simulink model "xPC_parker"  (Simulink 8.5)
settings: Solver=FixedStepDiscrete  StartTime=0.0  StopTime=inf  FixedStep=dts  RelTol=1e-3
InitFcn:
  | PARKER_DEPENDENCY
  | Parker_Multi_Axis_Init
  | Parker_ATI_Init
  | Parker_Home_Init
  | Parker_Davinci_Init
  | Parker_UDP_Init
  | Parker_LinIntPathPlan_Init
  | Parker_ScopeFormat_Init
  | Parker_magnetic_init
undefined symbols (not defined in the file): A, accel_filter_coeffs, ATI_torque_Nmm, B, counter_offset, DavinciFilterDen, DavinciFilterNum, DesiredPath, dt, dt_ENC, dt_trakstar, dts, dtudp, ENC_obs_filter_coeffs, encoder_counts, F, f_mag_desired_shape, filter_coeffs_bias, force_bias, forceDeadZone, FT_unbias_time, grav_vector, Home_in_TKbase, HOMING_dx, HOMING_num_joint, HOMING_tspan, HOMING_Vmov, inv_T, JOINT_Limits_Negative, JOINT_Limits_Postive, Kd, Ki_force, Kp, Kp_force, Kv_force, Low, N_acceleration, N_bias, N_ENC_obs_filter, N_obs_velocity, N_trakstar, N_velocity, Omega7IsLeftHanded, omni_scaling, PathPlanSpeed, pitch, quadrature_mode, R_FT2robot, R_omni, R_robot2TKbase, ResRateEpsilon, ResRateVelLimits, ResRateVelRatios, SafetyMargin, screw_pitch, torque_constant, trakstar_filter_coeffs, UDP_EN_Data2CMU, UDP_EN_DynAna, UDP_EN_VFRec ... (+6)
libraries: slrtlib x25, simulink x24, dspswit3 x15, xpcobsoletelib x15, xpcrtudplib x14, powerlib_meascontrol x3, xpcmeasurementcomputinglib x3, xpcconteclib x3
(part 2 of 3)

== system xPC_parker/Parker 404XR/Plant ==
  u : Inport
  "1STPORTB " : xpcmeasurementcomputinglib/Digital Input/PCI-DDA08 12   channel=[3 4 7]  port=C  chip=1  sampletime=dt  slot=-1
  CNT32-8M(PCI) Ch1 : xpcconteclib/Incremental Encoder/CNT32-8M(PCI)   Channel=1  OperationMode=2-phase Input Synchronous Clear Multiply by 4  DigitalFilter=No filtering  PulseInput=Differential line receiver input  Direction=Down in the clockwise direction/Up in the counterclockwise direction  InitialValue=counter_offset  LoadInitialValue=on  SampleTime=dt_ENC  PciSlot=-1  StartMethod=Model Start  StopMethod=Model Terminate  ZeroClearRising=off  ZeroClearFalling=off  ZeroClearMatch0=off  ZeroClearMatch1=off  PresetRising=off  PresetFalling=off  PresetMatch0=off  PresetMatch1=off  PresetValue=0  Match0Value=0  Match1Value=0  OutputSignalMatch0=off  OutputSignalMatch1=off  OutputSignalAbnormal=off  OutputSignalDigitalFilter=off  OutputSignalAlarm=off  OneShotDuration=10 microseconds  IndexEnable=Disable  IndexLogic=Positive (Active High)  EnableDigitalInput=off  EnableDigitalOutput=off  DigitalOutputInitialValue=None  DigitalOutputFinalValue=None
  CNT32-8M(PCI) Ch2 : xpcconteclib/Incremental Encoder/CNT32-8M(PCI)   Channel=2  OperationMode=2-phase Input Synchronous Clear Multiply by 4  DigitalFilter=No filtering  PulseInput=Differential line receiver input  Direction=Up in the clockwise direction/Down in the counterclockwise direction  InitialValue=counter_offset  LoadInitialValue=on  SampleTime=dt_ENC  PciSlot=-1  StartMethod=Model Start  StopMethod=Model Terminate  ZeroClearRising=off  ZeroClearFalling=off  ZeroClearMatch0=off  ZeroClearMatch1=off  PresetRising=off  PresetFalling=off  PresetMatch0=off  PresetMatch1=off  PresetValue=0  Match0Value=0  Match1Value=0  OutputSignalMatch0=off  OutputSignalMatch1=off  OutputSignalAbnormal=off  OutputSignalDigitalFilter=off  OutputSignalAlarm=off  OneShotDuration=10 microseconds  IndexEnable=Disable  IndexLogic=Positive (Active High)  EnableDigitalInput=off  EnableDigitalOutput=off  DigitalOutputInitialValue=None  DigitalOutputFinalValue=None
  CNT32-8M(PCI) Ch3 : xpcconteclib/Incremental Encoder/CNT32-8M(PCI)   Channel=3  OperationMode=2-phase Input Synchronous Clear Multiply by 4  DigitalFilter=No filtering  PulseInput=Differential line receiver input  Direction=Down in the clockwise direction/Up in the counterclockwise direction  InitialValue=counter_offset  LoadInitialValue=on  SampleTime=dt_ENC  PciSlot=-1  StartMethod=Model Start  StopMethod=Model Terminate  ZeroClearRising=off  ZeroClearFalling=off  ZeroClearMatch0=off  ZeroClearMatch1=off  PresetRising=off  PresetFalling=off  PresetMatch0=off  PresetMatch1=off  PresetValue=0  Match0Value=0  Match1Value=0  OutputSignalMatch0=off  OutputSignalMatch1=off  OutputSignalAbnormal=off  OutputSignalDigitalFilter=off  OutputSignalAlarm=off  OneShotDuration=10 microseconds  IndexEnable=Disable  IndexLogic=Positive (Active High)  EnableDigitalInput=off  EnableDigitalOutput=off  DigitalOutputInitialValue=None  DigitalOutputFinalValue=None
  Demux : Demux  Outputs=3
  Gain : Gain  Gain=-1
  Logical Operator : Logic  Operator=NOT  Inputs=1  AllPortsSameDT=off  OutDataTypeStr=boolean
  Mux : Mux  Inputs=3
  Mux1 : Mux  Inputs=3
  "PCI-DDA08 12 " : xpcmeasurementcomputinglib/D//A/PCI-DDA08 12   channel=[4 5 6]  range=[-10 -10 -10]  reset=[1 1 1]  initValue=[0 0 0]  sampletime=dt  pci_dev=-1
  counts : Outport
  LimitSW : Outport  Port=2
  tag scope: Scope_limit_SW=global
  wires:
  Demux/3 -> "PCI-DDA08 12 "/3
  Gain/1 -> "PCI-DDA08 12 "/2
  CNT32-8M(PCI) Ch3/1 -> Mux/3
  CNT32-8M(PCI) Ch2/1 -> Mux/2
  CNT32-8M(PCI) Ch1/1 -> Mux/1
  Demux/2 -> Gain/1
  Demux/1 -> "PCI-DDA08 12 "/1
  u/1 -> Demux/1
  "1STPORTB "/1 -> Mux1/1
  "1STPORTB "/2 -> Mux1/2
  "1STPORTB "/3 -> Mux1/3
  Mux/1 -> counts/1
  Mux1/1 -> Logical Operator/1
  Logical Operator/1 -> [Scope_limit_SW], LimitSW/1

== system xPC_parker/Scopes/Enabled Subsystem ==
  wrench : Inport
  p_cur : Inport  Port=2
  Enable : EnablePort
  Gain : Gain
  Gain1 : Gain
  "ft_Scope " : slrtlib/Displays and Logging/Scope   scopeno=26  scopetype=File  autostart=on  viewmode=Graphical redraw  formatstr='%15.6f'  grid=on  ylimits=[0,0]  nosamples=50000  noprepostsamples=0  interleave=1  triggermode=FreeRun  triggersignal=1  trigsignalfromport=off  triggerlevel=0.0  triggerslope=Either  triggerscope=1  triggersample=0  filename=Ft_<%%%>.dat  mode=Lazy  writesize=512  autorestart=on  dynamicfilemode=on  maxwritefilesize=512*1024^2
  "pc_Scope " : slrtlib/Displays and Logging/Scope   scopeno=27  scopetype=File  autostart=on  viewmode=Graphical redraw  formatstr='%15.6f'  grid=on  ylimits=[0,0]  nosamples=50000  noprepostsamples=0  interleave=1  triggermode=FreeRun  triggersignal=1  trigsignalfromport=off  triggerlevel=0.0  triggerslope=Either  triggerscope=1  triggersample=0  filename=Pc_<%%%>.dat  mode=Lazy  writesize=512  autorestart=on  dynamicfilemode=on  maxwritefilesize=512*1024^2
  wires:
  wrench/1 -> Gain1/1
  p_cur/1 -> Gain/1
  Gain/1 -> "pc_Scope "/1
  Gain1/1 -> "ft_Scope "/1

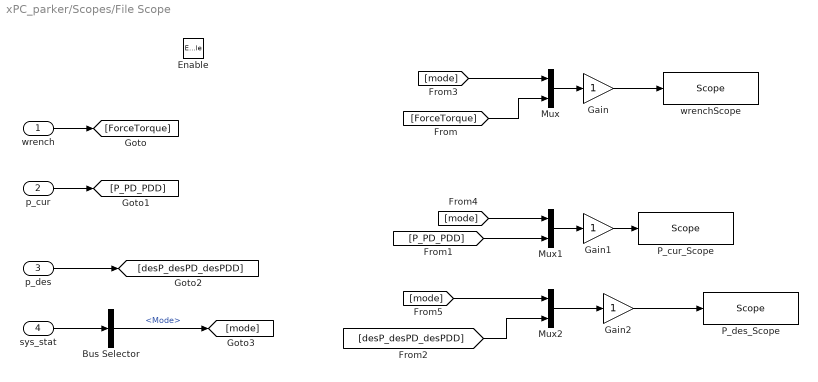
== system xPC_parker/Scopes/File Scope ==
  wrench : Inport
  p_cur : Inport  Port=2
  p_des : Inport  Port=3
  sys_stat : Inport  Port=4
  Enable : EnablePort
  Bus Selector : BusSelector  OutputSignals=Mode
  Gain : Gain
  Gain1 : Gain
  Gain2 : Gain
  Mux : Mux  Inputs=2
  Mux1 : Mux  Inputs=2
  Mux2 : Mux  Inputs=2
  P_cur_Scope : slrtlib/Displays and Logging/Scope   scopeno=13  scopetype=File  autostart=on  viewmode=Numerical  formatstr=forceFormat  grid=on  ylimits=[0,0]  nosamples=50000  noprepostsamples=0  interleave=1  triggermode=FreeRun  triggersignal=1  trigsignalfromport=off  triggerlevel=0.0  triggerslope=Either  triggerscope=1  triggersample=0  filename=Cur_<%%%>.dat  mode=Lazy  writesize=512  autorestart=on  dynamicfilemode=on  maxwritefilesize=512*1024^2
  P_des_Scope : slrtlib/Displays and Logging/Scope   scopeno=14  scopetype=File  autostart=on  viewmode=Numerical  formatstr=forceFormat  grid=on  ylimits=[0,0]  nosamples=50000  noprepostsamples=0  interleave=1  triggermode=FreeRun  triggersignal=1  trigsignalfromport=off  triggerlevel=0.0  triggerslope=Either  triggerscope=1  triggersample=0  filename=Des_<%%%>.dat  mode=Lazy  writesize=512  autorestart=on  dynamicfilemode=on  maxwritefilesize=512*1024^2
  wrenchScope : slrtlib/Displays and Logging/Scope   scopeno=16  scopetype=File  autostart=on  viewmode=Numerical  formatstr=forceFormat  grid=on  ylimits=[0,0]  nosamples=50000  noprepostsamples=0  interleave=1  triggermode=FreeRun  triggersignal=1  trigsignalfromport=off  triggerlevel=0.0  triggerslope=Either  triggerscope=1  triggersample=0  filename=We_<%%%>.dat  mode=Lazy  writesize=512  autorestart=on  dynamicfilemode=on  maxwritefilesize=512*1024^2
  wires:
  wrench/1 -> [ForceTorque]
  p_cur/1 -> [P_PD_PDD]
  p_des/1 -> [desP_desPD_desPDD]
  sys_stat/1 -> Bus Selector/1
  Bus Selector/1 -> [mode]  "<Mode>"
  Mux/1 -> Gain/1
  [ForceTorque] -> Mux/2
  [mode] -> Mux/1
  Mux1/1 -> Gain1/1
  [mode] -> Mux1/1
  [P_PD_PDD] -> Mux1/2
  Mux2/1 -> Gain2/1
  [mode] -> Mux2/1
  [desP_desPD_desPDD] -> Mux2/2
  Gain/1 -> wrenchScope/1
  Gain1/1 -> P_cur_Scope/1
  Gain2/1 -> P_des_Scope/1

== system xPC_parker/Scopes/MTM_convert_for_scope ==
  In : Inport
  Bus Selector1 : BusSelector  OutputSignals=MSG_Type,position,orientation (quat),MTM_time,Delay
  Gain : Gain
  Mux : Mux  Inputs=5
  Out : Outport
  wires:
  Mux/1 -> Gain/1
  Bus Selector1/1 -> Mux/1  "<MSG_Type>"
  Bus Selector1/2 -> Mux/2  "<position>"
  In/1 -> Bus Selector1/1
  Bus Selector1/3 -> Mux/3  "<orientation (quat)>"
  Bus Selector1/4 -> Mux/4  "<MTM_time>"
  Bus Selector1/5 -> Mux/5  "<Delay>"
  Gain/1 -> Out/1

== system xPC_parker/Scopes/Omni_convert_for_scope ==
  In : Inport
  Bus Selector1 : BusSelector  OutputSignals=enable,position,orientation (quat)
  Mux : Mux  Inputs=3
  Out : Outport
  wires:
  Bus Selector1/3 -> Mux/3  "<orientation (quat)>"
  Bus Selector1/2 -> Mux/2  "<position>"
  Mux/1 -> Out/1
  In/1 -> Bus Selector1/1
  Bus Selector1/1 -> Mux/1  "<enable>"

== system xPC_parker/Scopes/Path_convert_for_scope ==
  In : Inport
  Bus Selector1 : BusSelector  OutputSignals=dState,cState,x,t,s
  Mux : Mux  Inputs=5
  Out : Outport
  wires:
  In/1 -> Bus Selector1/1
  Mux/1 -> Out/1
  Bus Selector1/5 -> Mux/5  "<s>"
  Bus Selector1/1 -> Mux/1  "<dState>"
  Bus Selector1/3 -> Mux/3  "<x>"
  Bus Selector1/2 -> Mux/2  "<cState>"
  Bus Selector1/4 -> Mux/4  "<t>"

== system xPC_parker/Scopes/UDP VF Record Data ==
  p_cur : Inport
  cmd : Inport  Port=2
  Enable : EnablePort
  Bus Selector1 : BusSelector  OutputSignals=position,velocity
  Demux1 : Demux  Outputs=11
  Digital Clock : DigitalClock  SampleTime=dtudp
  Mux3 : Mux  Inputs=5
  Pack : xpcobsoletelib/Utilities/Pack   datatypes={'double' 'double' 'double' 'double' 'double' 'double' 'double' 'double' 'double' 'double' 'double'}  byteAlign=1
  Parker_VF_Record : xpcrtudplib/Legacy UDP/Send   ipAddress=255.255.255.255  ipPort=UDP_PORT_DataVFRec  localPort=-1  vblLen=off  sampletime=dtUDP_Data
  Rate Transition2 : RateTransition  OutPortSampleTime=dtUDP_Data
  STOP : Constant
  wires:
  Pack/1 -> Parker_VF_Record/1
  Mux3/1 -> Rate Transition2/1
  Rate Transition2/1 -> Demux1/1
  Demux1/1 -> Pack/1
  Demux1/2 -> Pack/2
  Demux1/3 -> Pack/3
  Demux1/4 -> Pack/4
  Demux1/5 -> Pack/5
  Demux1/6 -> Pack/6
  Demux1/7 -> Pack/7
  Demux1/8 -> Pack/8
  Demux1/9 -> Pack/9
  Demux1/10 -> Pack/10
  Demux1/11 -> Pack/11
  STOP/1 -> Mux3/5
  p_cur/1 -> Bus Selector1/1
  cmd/1 -> Mux3/3
  Bus Selector1/1 -> Mux3/1  "<position>"
  Bus Selector1/2 -> Mux3/2  "<velocity>"
  Digital Clock/1 -> Mux3/4

== system xPC_parker/Trajectory Planner/DaVinci MTM port: 2 ==
  pc : Inport
  force : Inport  Port=2
  Hybrid_EN : Inport  Port=3
  Enable : EnablePort  StatesWhenEnabling=reset
  Bus Selector : BusSelector  OutputSignals=x_cmd,v_cmd
  DaVinci MTM : Subsystem
  Davinci Task Ref : Subsystem  TreatAsAtomicUnit=on
  UDP_feedback_to_MTM : Subsystem
  x_cmd : Outport
  MTM Read : Outport  Port=2
  v_cmd : Outport  Port=3
  wires:
  DaVinci MTM/1(MTM) -> MTM Read/1, Davinci Task Ref/1(MTM), UDP_feedback_to_MTM/1(MTM)
  pc/1 -> UDP_feedback_to_MTM/4(pc), Davinci Task Ref/2(x_cmd_prev)
  Davinci Task Ref/1(traj) -> UDP_feedback_to_MTM/2(traj), Bus Selector/1
  Bus Selector/1 -> x_cmd/1  "<x_cmd>"
  force/1 -> UDP_feedback_to_MTM/3(force)
  Bus Selector/2 -> v_cmd/1  "<v_cmd>"
  Hybrid_EN/1 -> Davinci Task Ref/3(Hybrid_EN)

== system xPC_parker/Trajectory Planner/Homing ==
  q_cur,Sw : Inport
  Enable : EnablePort  StatesWhenEnabling=reset
  A Delay : UnitDelay  InitialCondition=zeros(HOMING_num_joint,4)  SampleTime=dt
  Bus Selector : BusSelector  OutputSignals=LimitSW
  Bus Selector1 : BusSelector  OutputSignals=position
  Homing Procedure : MATLAB Function  TreatAsAtomicUnit=on
  Mux : Mux  Inputs=3
  N-Sample Switch : dspswit3/N-Sample Switch  N=1  reset=off  TriggerType=Rising edge  Ts=dt
  V_mov : Constant  Value=HOMING_Vmov  SampleTime=dt
  dt : Constant  Value=dt  SampleTime=dt
  home_pos : Constant  Value=HOMING_dx  SampleTime=dt
  homing ready delay : UnitDelay  SampleTime=dt
  lsf delay : UnitDelay  InitialCondition=ones(HOMING_num_joint,1)  SampleTime=dt
  qdes Delay : UnitDelay  InitialCondition=zeros(HOMING_num_joint,1)  SampleTime=dt
  status delay : UnitDelay  SampleTime=dt
  tspan : Constant  Value=HOMING_tspan  SampleTime=dt
  Encoder Reset : Outport
  q,qd,qdd_des : Outport  Port=2
  Homing stat : Outport  Port=3
  wires:
  Homing Procedure/1(q_des) -> qdes Delay/1, Mux/1
  Bus Selector/1 -> Homing Procedure/5(switches)  "<LimitSW>"
  Homing Procedure/4(ready) -> homing ready delay/1, Homing stat/1
  homing ready delay/1 -> Homing Procedure/7(stop_flag)
  dt/1 -> Homing Procedure/1(dt)
  qdes Delay/1 -> N-Sample Switch/2
  N-Sample Switch/1 -> Homing Procedure/6(q_prev)
  Bus Selector1/1 -> Homing Procedure/10(q_cur), N-Sample Switch/1  "<position>"
  home_pos/1 -> Homing Procedure/4(home_pos)
  Homing Procedure/5(A_out) -> A Delay/1
  A Delay/1 -> Homing Procedure/8(A_in)
  Homing Procedure/6(cur_status) -> status delay/1
  status delay/1 -> Homing Procedure/9(prev_status)
  Homing Procedure/7(reset) -> Encoder Reset/1
  Homing Procedure/8(lsf_out) -> lsf delay/1
  lsf delay/1 -> Homing Procedure/11(lsf_in)
  Homing Procedure/2(qd_des) -> Mux/2
  Homing Procedure/3(qdd_des) -> Mux/3
  Mux/1 -> q,qd,qdd_des/1
  q_cur,Sw/1 -> [q_cur]
  [q_cur] -> Bus Selector/1
  [q_cur] -> Bus Selector1/1
  tspan/1 -> Homing Procedure/2(tspan)
  V_mov/1 -> Homing Procedure/3(V_mov)

== system xPC_parker/Trajectory Planner/Omega7 ==
  note: This version works with Ellie's omega7 code 2015/7/21
  pc : Inport
  force : Inport  Port=2
  Enable : EnablePort  StatesWhenEnabling=reset
  Bus Creator : BusCreator  Inputs=3
  Constant : Constant  Value=0.3
  Constant1 : Constant  Value=Omega7IsLeftHanded
  Discrete Filter : DiscreteFilter  Numerator=DavinciFilterNum  Denominator=DavinciFilterDen
  Discrete Filter1 : DiscreteFilter  Numerator=DavinciFilterNum  Denominator=DavinciFilterDen
  Feedback_to_omega7 : Subsystem
  MATLAB Function : MATLAB Function  TreatAsAtomicUnit=on
  Mux1 : Mux  Inputs=3
  Mux2 : Mux
  Omni Task Ref : Subsystem  TreatAsAtomicUnit=on
  Rate Transition3 : RateTransition  OutPortSampleTime=dt
  Receive : xpcrtudplib/Legacy UDP/Receive   ipAddress=000.000.000.000  ipPort=26999  width=72  vblLen=on  sampletime=dtOmega7
  Terminator : Terminator
  Unpack : xpcobsoletelib/Utilities/Unpack   dimensions={1,1,1,1,1,1,1,1,1}  datatypes={'double' 'double' 'double' 'double' 'double' 'double' 'double' 'double' 'double'}  byteAlign=1
  m to mm : Gain  Gain=1000
  x_cmd : Outport
  Omni Read : Outport  Port=2
  v_cmd : Outport  Port=3
  wires:
  Receive/1 -> Unpack/1
  Receive/2 -> Terminator/1
  Bus Creator/1 -> Rate Transition3/1
  Mux1/1 -> m to mm/1  "position"
  Mux2/1 -> Discrete Filter1/1  "orientation (quat)"
  Omni Task Ref/1(x_cmd) -> x_cmd/1
  Rate Transition3/1 -> Omni Task Ref/1(Omni), Omni Read/1
  pc/1 -> Omni Task Ref/2(x_cmd_prev)
  force/1 -> Feedback_to_omega7/1(force)
  Omni Task Ref/2(v_cmd) -> v_cmd/1
  Unpack/1 -> MATLAB Function/1(online)  "online"
  Unpack/2 -> MATLAB Function/2(GP)  "gripper angle"
  Unpack/3 -> Mux1/1
  Unpack/4 -> Mux1/2
  Unpack/5 -> Mux1/3
  Unpack/9 -> Mux2/4
  Unpack/6 -> Mux2/1
  Unpack/7 -> Mux2/2
  Unpack/8 -> Mux2/3
  MATLAB Function/1(enable) -> Bus Creator/1  "enable"
  Constant/1 -> MATLAB Function/3(GP_thresh)
  m to mm/1 -> Discrete Filter/1  "position"
  Constant1/1 -> MATLAB Function/4(LeftHand)
  Discrete Filter/1 -> Bus Creator/2  "position"
  Discrete Filter1/1 -> Bus Creator/3  "orientation (quat)"

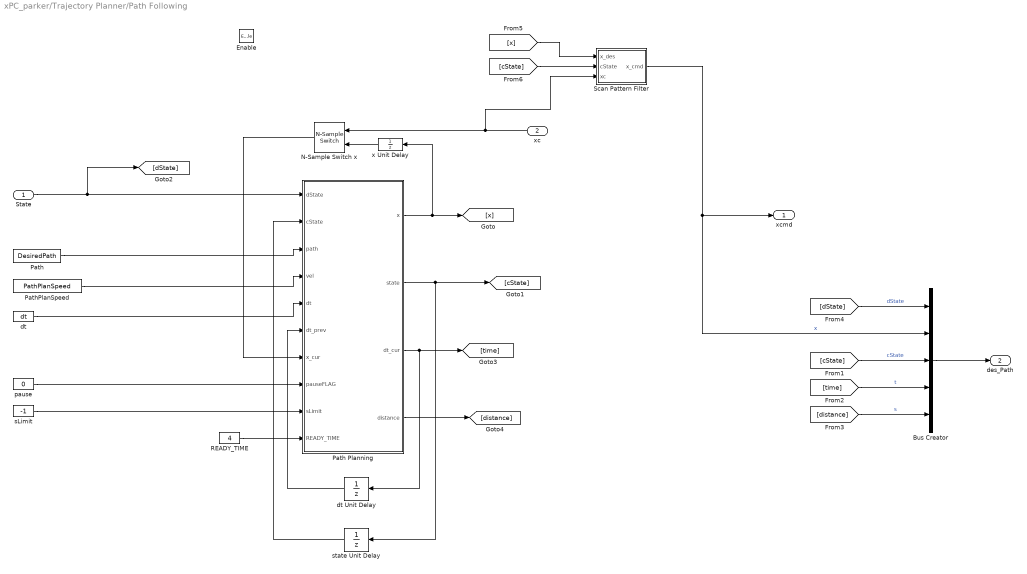
== system xPC_parker/Trajectory Planner/Path Following ==
  State : Inport
  xc : Inport  Port=2
  Enable : EnablePort  StatesWhenEnabling=reset
  Bus Creator : BusCreator  Inputs=5
  N-Sample Switch x : dspswit3/N-Sample Switch  N=1  reset=off  TriggerType=Non-zero sample  Ts=dt
  Path : Constant  Value=DesiredPath
  Path Planning : MATLAB Function  TreatAsAtomicUnit=on
  PathPlanSpeed : Constant  Value=PathPlanSpeed
  READY_TIME : Constant  Value=4
  Scan Pattern Filter : MATLAB Function  TreatAsAtomicUnit=on
  dt : Constant  Value=dt
  dt Unit Delay : UnitDelay  SampleTime=-1
  pause : Constant  Value=0
  sLimit : Constant  Value=-1
  state Unit Delay : UnitDelay  InitialCondition=1  SampleTime=-1
  x Unit Delay : UnitDelay  InitialCondition=[0;0;0]  SampleTime=-1
  xcmd : Outport
  des_Path : Outport  Port=2
  wires:
  Path Planning/2(state) -> [cState], state Unit Delay/1
  Path Planning/1(x) -> x Unit Delay/1, [x]
  Path/1 -> Path Planning/3(path)
  PathPlanSpeed/1 -> Path Planning/4(vel)
  State/1 -> [dState], Path Planning/1(dState)
  dt Unit Delay/1 -> Path Planning/6(dt_prev)
  state Unit Delay/1 -> Path Planning/2(cState)
  Path Planning/3(dt_cur) -> [time], dt Unit Delay/1
  dt/1 -> Path Planning/5(dt)
  Path Planning/4(distance) -> [distance]
  N-Sample Switch x/1 -> Path Planning/7(x_cur)
  x Unit Delay/1 -> N-Sample Switch x/2
  xc/1 -> Scan Pattern Filter/3(xc), N-Sample Switch x/1
  pause/1 -> Path Planning/8(pauseFLAG)
  sLimit/1 -> Path Planning/9(sLimit)
  [dState] -> Bus Creator/1  "dState"
  Scan Pattern Filter/1(x_cmd) -> Bus Creator/2, xcmd/1  "x"
  [cState] -> Bus Creator/3  "cState"
  [time] -> Bus Creator/4  "t"
  [distance] -> Bus Creator/5  "s"
  Bus Creator/1 -> des_Path/1
  READY_TIME/1 -> Path Planning/10(READY_TIME)
  [x] -> Scan Pattern Filter/1(x_des)
  [cState] -> Scan Pattern Filter/2(cState)

== system xPC_parker/Trajectory Planner/Quintic Polynomial ==
  In1 : Inport
  Enable : EnablePort  StatesWhenEnabling=reset
  5th Order Polynomial : Subsystem
  Bus Selector : BusSelector  OutputSignals=position
  Get_Initial_Condition : Subsystem
  Manual : Constant  Value=0
  Multiport Switch : MultiPortSwitch  DataPortOrder=Zero-based contiguous  Inputs=2
  Mux : Mux  Inputs=2
  "Scope " : slrtlib/Displays and Logging/Scope   scopeno=22  scopetype=Target  autostart=on  viewmode=Numerical  formatstr='%15.6f'  grid=on  ylimits=[0,0]  nosamples=250  noprepostsamples=0  interleave=1  triggermode=FreeRun  triggersignal=1  trigsignalfromport=off  triggerlevel=0.0  triggerslope=Either  triggerscope=1  triggersample=0  filename=data.dat  mode=Lazy  writesize=512  autorestart=off  dynamicfilemode=off  maxwritefilesize=512*1024^2
  enable : Constant
  q_des : Constant  Value=[0;0;0]
  trigger detection : Subsystem
  "p, pd, pdd" : Outport  InitialOutput=zeros(9,1)
  QuinticRecord : Outport  Port=2  InitialOutput=0
  wires:
  enable/1 -> 5th Order Polynomial/3(enable)
  In1/1 -> Bus Selector/1
  Bus Selector/1 -> 5th Order Polynomial/2(q curr), Get_Initial_Condition/1(q_cur)  "<position>"
  5th Order Polynomial/1(q,qd,qdd) -> "p, pd, pdd"/1
  Multiport Switch/1 -> 5th Order Polynomial/1(q des)
  q_des/1 -> Multiport Switch/3
  Get_Initial_Condition/1(Initial) -> Multiport Switch/2
  5th Order Polynomial/2(RecordFlag) -> QuinticRecord/1
  Manual/1 -> trigger detection/1(trig)
  trigger detection/1(enable) -> Mux/2, Multiport Switch/1
  trigger detection/2(count) -> Mux/1
  Mux/1 -> "Scope "/1

== system xPC_parker/Trajectory Planner/Task Enable Logic ==
  note: This Manual Enable Control is not often used.
      | You Do not need this for most of the time,
      | unless you are sure you need this for some very particular experiments.
  Omni : Inport
  MTM : Inport  Port=2
  PATH : Inport  Port=3
  Add : Sum  Inputs=++++
  Bus Selector : BusSelector  OutputSignals=enable
  Bus Selector1 : BusSelector  OutputSignals=MSG_Type
  Bus Selector2 : BusSelector  OutputSignals=cState
  MATLAB Function : MATLAB Function  TreatAsAtomicUnit=on
  Manual Enable : Constant  Value=0
  PathPlannerLogic : Subsystem
  Unit Delay : UnitDelay  SampleTime=-1
  TeleEN : Outport
  wires:
  Omni/1 -> Bus Selector/1
  MTM/1 -> Bus Selector1/1
  Bus Selector/1 -> Add/1  "<enable>"
  Bus Selector1/1 -> MATLAB Function/1(MSG_TYPE)  "<MSG_Type>"
  MATLAB Function/1(Task_EN) -> Add/2
  Add/1 -> Unit Delay/1
  Unit Delay/1 -> TeleEN/1
  PATH/1 -> Bus Selector2/1
  Bus Selector2/1 -> PathPlannerLogic/1(cState)  "<cState>"
  PathPlannerLogic/1(TASK_EN) -> Add/3
  Manual Enable/1 -> Add/4

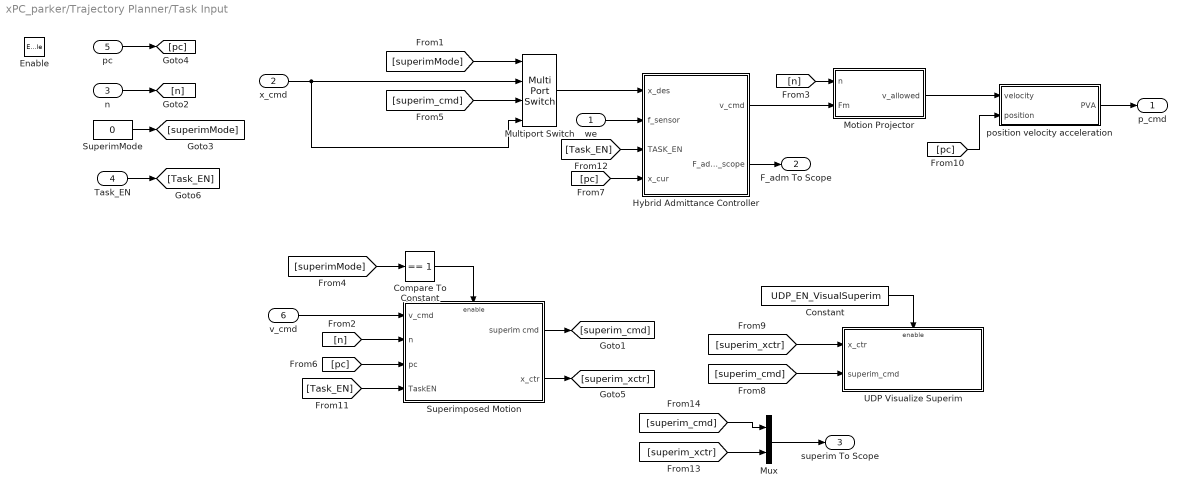
== system xPC_parker/Trajectory Planner/Task Input ==
  we : Inport
  x_cmd : Inport  Port=2
  n : Inport  Port=3
  Task_EN : Inport  Port=4
  pc : Inport  Port=5
  v_cmd : Inport  Port=6
  Enable : EnablePort  StatesWhenEnabling=reset
  Compare To Constant : simulink/Logic and Bit Operations/Compare To Constant  relop===  const=1  OutDataTypeStr=boolean
  Constant : Constant  Value=UDP_EN_VisualSuperim
  Hybrid Admittance Controller : Subsystem
  Motion Projector : Subsystem  TreatAsAtomicUnit=on
  Multiport Switch : MultiPortSwitch  DataPortOrder=Zero-based contiguous  Inputs=2  DataPortForDefault=Additional data port
  Mux : Mux  Inputs=2
  SuperimMode : Constant  Value=0
  Superimposed Motion : Subsystem
  UDP Visualize Superim : Subsystem
  position velocity acceleration : Subsystem
  p_cmd : Outport
  F_adm To Scope : Outport  Port=2
  superim To Scope : Outport  Port=3
  wires:
  we/1 -> Hybrid Admittance Controller/2(f_sensor)
  Hybrid Admittance Controller/2(F_adm_scope) -> F_adm To Scope/1
  position velocity acceleration/1(PVA) -> p_cmd/1
  Hybrid Admittance Controller/1(v_cmd) -> Motion Projector/2(Fm)
  Motion Projector/1(v_allowed) -> position velocity acceleration/1(velocity)
  Constant/1 -> UDP Visualize Superim/Enable
  n/1 -> [n]
  [n] -> Superimposed Motion/2(n)
  [n] -> Motion Projector/1(n)
  v_cmd/1 -> Superimposed Motion/1(v_cmd)
  Superimposed Motion/1(superim cmd) -> [superim_cmd]
  x_cmd/1 -> Multiport Switch/2, Multiport Switch/4
  SuperimMode/1 -> [superimMode]
  [superimMode] -> Multiport Switch/1
  Multiport Switch/1 -> Hybrid Admittance Controller/1(x_des)
  [superimMode] -> Compare To Constant/1
  Compare To Constant/1 -> Superimposed Motion/Enable
  [superim_cmd] -> Multiport Switch/3
  pc/1 -> [pc]
  [pc] -> Superimposed Motion/3(pc)
  [pc] -> Hybrid Admittance Controller/4(x_cur)
  Superimposed Motion/2(x_ctr) -> [superim_xctr]
  [superim_cmd] -> UDP Visualize Superim/2(superim_cmd)
  [superim_xctr] -> UDP Visualize Superim/1(x_ctr)
  [pc] -> position velocity acceleration/2(position)
  Task_EN/1 -> [Task_EN]
  [Task_EN] -> Superimposed Motion/4(TaskEN)
  [Task_EN] -> Hybrid Admittance Controller/3(TASK_EN)
  Mux/1 -> superim To Scope/1
  [superim_xctr] -> Mux/2
  [superim_cmd] -> Mux/1

== system xPC_parker/Trajectory Planner/safety check ==
  In1 : Inport
  Unit Delay2 : UnitDelay  InitialCondition=zeros(9,1)  SampleTime=-1
  Unit Delay3 : UnitDelay  SampleTime=-1
  false detection : MATLAB Function  TreatAsAtomicUnit=on
  Out : Outport
  error_flag : Outport  Port=2
  wires:
  false detection/1(pva_allowed) -> Unit Delay2/1, Out/1
  Unit Delay2/1 -> false detection/2(pva_prev)
  In1/1 -> false detection/1(pva_cmd)
  Unit Delay3/1 -> false detection/3(error_prev)
  false detection/2(error_flag) -> Unit Delay3/1, error_flag/1

== system xPC_parker/Force Sensor/Contact_Estimation/Force Contact Filter ==
  V_in : Inport  SampleTime=dts
  Discrete FIR Filter : DiscreteFir  CoefSource=Input port  SampleTime=dts  AccumDataTypeStr=Inherit: Same as product output
  Gain : Gain  Gain=1/25  SampleTime=dts
  filter_coeffs : Constant  Value=ones(25,1)  SampleTime=dt
  V_Out : Outport  SampleTime=dts
  wires:
  Gain/1 -> V_Out/1
  filter_coeffs/1 -> Discrete FIR Filter/2
  Discrete FIR Filter/1 -> Gain/1
  V_in/1 -> Discrete FIR Filter/1

== system xPC_parker/Force Sensor/Contact_Estimation/Surf Norm Filter ==
  V_in : Inport  SampleTime=dts
  Discrete FIR Filter : DiscreteFir  CoefSource=Input port  SampleTime=dts  AccumDataTypeStr=Inherit: Same as product output
  Gain : Gain  Gain=1/100  SampleTime=dts
  filter_coeffs : Constant  Value=ones(100,1)  SampleTime=dt
  V_Out : Outport  SampleTime=dts
  wires:
  Gain/1 -> V_Out/1
  filter_coeffs/1 -> Discrete FIR Filter/2
  Discrete FIR Filter/1 -> Gain/1
  V_in/1 -> Discrete FIR Filter/1

== system xPC_parker/Force Sensor/Data_to_CMU/UDP ==
  In1 : Inport
  In2 : Inport  Port=2
  In3 : Inport  Port=3
  Enable : EnablePort
  Demux2 : Demux  Outputs=8
  Digital Clock : DigitalClock  SampleTime=dtudp
  Mux2 : Mux
  Pack1 : xpcobsoletelib/Utilities/Pack   datatypes={'double' 'double' 'double' 'double' 'double' 'double' 'double' 'double'}  byteAlign=1
  Parker_Send_CMU : xpcrtudplib/Legacy UDP/Send   ipAddress=255.255.255.255  ipPort=UDP_PORT_DataSend2CMU  localPort=-1  vblLen=off  sampletime=dtUDP_CMU
  Rate Transition1 : RateTransition  OutPortSampleTime=dtUDP_CMU
  Receive_from_CMU : xpcrtudplib/Legacy UDP/Receive   ipAddress=000.000.000.000  ipPort=UDP_PORT_DataRecvFromCMU  width=8*1  vblLen=on  sampletime=dtUDP_CMU
  Sum1 : Sum  Inputs=|+-  SampleTime=dts
  Terminator1 : Terminator
  Unpack1 : xpcobsoletelib/Utilities/Unpack   dimensions={1}  datatypes={'double'}  byteAlign=1
  sec to ms : Gain  Gain=1000
  delay in ms : Outport  InitialOutput=9999999
  wires:
  Mux2/1 -> Rate Transition1/1
  Pack1/1 -> Parker_Send_CMU/1
  Rate Transition1/1 -> Demux2/1
  Demux2/1 -> Pack1/1
  Demux2/2 -> Pack1/2
  Demux2/4 -> Pack1/4
  Demux2/3 -> Pack1/3
  Demux2/5 -> Pack1/5
  Demux2/6 -> Pack1/6
  Demux2/7 -> Pack1/7
  Receive_from_CMU/2 -> Terminator1/1
  Receive_from_CMU/1 -> Unpack1/1
  Sum1/1 -> sec to ms/1
  Demux2/8 -> Pack1/8
  Unpack1/1 -> Sum1/2
  Digital Clock/1 -> Mux2/4, Sum1/1
  sec to ms/1 -> delay in ms/1
  In1/1 -> Mux2/1
  In2/1 -> Mux2/2
  In3/1 -> Mux2/3

== system xPC_parker/Hybrid Motion PD Inverse Dynamics/Surf Norm Command/Conflict Check ==
  note: This block is to prevent the following case happening:
      | Let's say the motion command is given in (x,y) plane;
      | However the robot is stopped by an obticle in x direction;
      | So now the force control direction will be possibly in (x,y) plane;
      | i.e. the meaningful command will be all filtered out.
      | We do not want this, so we want to artificially change the force control direction such that it is not perpendicular to Z
  surf_norm : Inport
  default : Inport  Port=2
  Angle Compensation : Subsystem  TreatAsAtomicUnit=on
  Out1 : Outport
  wires:
  Angle Compensation/1(Out1) -> Out1/1
  default/1 -> Angle Compensation/1(default_n)
  surf_norm/1 -> Angle Compensation/2(surf_norm)

== system xPC_parker/Parker 404XR/Count to Position/Accel Filter ==
  note: current velocity
  velocity : Inport
  Discrete Derivative1 : simulink/Discrete/Discrete Derivative  gainval=1.0  ICPrevScaledInput=0.0  InputProcessing=Inherited  OutMin=[]  OutMax=[]  OutDataType=sfix(16)  OutScaling=2^-10  DoSatur=off
  Discrete FIR Filter : DiscreteFir  CoefSource=Input port  AccumDataTypeStr=Inherit: Same as product output
  Gain : Gain  Gain=1/N_acceleration
  vel_filter_coeffs : Constant  Value=accel_filter_coeffs
  accel_out : Outport
  wires:
  Discrete FIR Filter/1 -> Gain/1
  vel_filter_coeffs/1 -> Discrete FIR Filter/2
  Gain/1 -> accel_out/1
  velocity/1 -> Discrete Derivative1/1
  Discrete Derivative1/1 -> Discrete FIR Filter/1

== system xPC_parker/Parker 404XR/Count to Position/Position Filter observer ==
  note: current velocity
  current_position : Inport
  Discrete FIR Filter : DiscreteFir  CoefSource=Input port  AccumDataTypeStr=Inherit: Same as product output
  Gain : Gain  Gain=1/N_ENC_obs_filter
  encoder obsever filter : Constant  Value=ENC_obs_filter_coeffs
  vel_out : Outport
  wires:
  current_position/1 -> Discrete FIR Filter/1
  Gain/1 -> vel_out/1
  encoder obsever filter/1 -> Discrete FIR Filter/2
  Discrete FIR Filter/1 -> Gain/1

== system xPC_parker/Parker 404XR/Count to Position/Position Filter observer1 ==
  note: current velocity
  current_position : Inport
  Discrete FIR Filter : DiscreteFir  CoefSource=Input port  AccumDataTypeStr=Inherit: Same as product output
  Gain : Gain  Gain=1/N_ENC_obs_filter
  encoder obsever filter : Constant  Value=ENC_obs_filter_coeffs
  vel_out : Outport
  wires:
  Discrete FIR Filter/1 -> Gain/1
  encoder obsever filter/1 -> Discrete FIR Filter/2
  Gain/1 -> vel_out/1
  current_position/1 -> Discrete FIR Filter/1

== system xPC_parker/Parker 404XR/Count to Position/Velocity Filter ==
  note: current velocity
  current_position : Inport
  Discrete Derivative : simulink/Discrete/Discrete Derivative  gainval=1.0  ICPrevScaledInput=0.0  InputProcessing=Inherited  OutMin=[]  OutMax=[]  OutDataType=sfix(16)  OutScaling=2^-10  DoSatur=off
  Discrete FIR Filter : DiscreteFir  CoefSource=Input port  AccumDataTypeStr=Inherit: Same as product output
  Gain : Gain  Gain=1/N_velocity
  vel_filter_coeffs : Constant  Value=vel_filter_coeffs
  vel_out : Outport
  wires:
  current_position/1 -> Discrete Derivative/1
  Discrete Derivative/1 -> Discrete FIR Filter/1
  Gain/1 -> vel_out/1
  vel_filter_coeffs/1 -> Discrete FIR Filter/2
  Discrete FIR Filter/1 -> Gain/1

== system xPC_parker/Parker 404XR/Count to Position/Velocity Filter observer ==
  note: current velocity
  current_position : Inport
  Discrete Derivative : simulink/Discrete/Discrete Derivative  gainval=1.0  ICPrevScaledInput=0.0  InputProcessing=Inherited  OutMin=[]  OutMax=[]  OutDataType=sfix(16)  OutScaling=2^-10  DoSatur=off
  Discrete FIR Filter : DiscreteFir  CoefSource=Input port  AccumDataTypeStr=Inherit: Same as product output
  Gain : Gain  Gain=1/N_obs_velocity
  vel_filter_coeffs : Constant  Value=vel_obs_filter_coeffs
  vel_out : Outport
  wires:
  Discrete FIR Filter/1 -> Gain/1
  vel_filter_coeffs/1 -> Discrete FIR Filter/2
  Gain/1 -> vel_out/1
  Discrete Derivative/1 -> Discrete FIR Filter/1
  current_position/1 -> Discrete Derivative/1

== system xPC_parker/Parker 404XR/Magnetic Tracker 125 Hz/process trak1 ==
  raw : Inport
  Filter1 : Subsystem
  Gain : Gain  Gain=[25.4 25.4 25.4 1 1 1]  SampleTime=dt_trakstar
  trakstar_to_pose : MATLAB Function  TreatAsAtomicUnit=on
  sensor_pose : Outport
  wires:
  Gain/1 -> Filter1/1(in)
  Filter1/1(out) -> trakstar_to_pose/1(u)
  raw/1 -> Gain/1
  trakstar_to_pose/1(sensor) -> sensor_pose/1

== system xPC_parker/Parker 404XR/Magnetic Tracker 125 Hz/process trak2 ==
  raw : Inport
  Filter1 : Subsystem
  Gain : Gain  Gain=[25.4 25.4 25.4 1 1 1]  SampleTime=dt_trakstar
  trakstar_to_pose : MATLAB Function  TreatAsAtomicUnit=on
  sensor_pose : Outport
  wires:
  trakstar_to_pose/1(sensor) -> sensor_pose/1
  raw/1 -> Gain/1
  Filter1/1(out) -> trakstar_to_pose/1(u)
  Gain/1 -> Filter1/1(in)

== system xPC_parker/Parker 404XR/Magnetic Tracker 125 Hz/process trak3 ==
  raw : Inport
  Filter1 : Subsystem
  Gain : Gain  Gain=[25.4 25.4 25.4 1 1 1]  SampleTime=dt_trakstar
  trakstar_to_pose : MATLAB Function  TreatAsAtomicUnit=on
  sensor_pose : Outport
  wires:
  Gain/1 -> Filter1/1(in)
  Filter1/1(out) -> trakstar_to_pose/1(u)
  raw/1 -> Gain/1
  trakstar_to_pose/1(sensor) -> sensor_pose/1

== system xPC_parker/Parker 404XR/Magnetic Tracker 125 Hz/process trak4 ==
  raw : Inport
  Filter1 : Subsystem
  Gain : Gain  Gain=[25.4 25.4 25.4 1 1 1]  SampleTime=dt_trakstar
  trakstar_to_pose : MATLAB Function  TreatAsAtomicUnit=on
  sensor_pose : Outport
  wires:
  trakstar_to_pose/1(sensor) -> sensor_pose/1
  raw/1 -> Gain/1
  Filter1/1(out) -> trakstar_to_pose/1(u)
  Gain/1 -> Filter1/1(in)

== system xPC_parker/Trajectory Planner/DaVinci MTM port: 2/DaVinci MTM ==
  Bus Creator1 : BusCreator  Inputs=8
  Discrete Derivative : simulink/Discrete/Discrete Derivative  gainval=1.0  ICPrevScaledInput=0.0  InputProcessing=Inherited  OutMin=[]  OutMax=[]  OutDataType=fixdt(1, 16)  OutScaling=2^-10  DoSatur=off
  Discrete Filter{,1..3} (4 alike) : DiscreteFilter  Numerator=DavinciFilterNum  Denominator=DavinciFilterDen
  MTM Filter : Subsystem
  Mux1 : Mux  Inputs=6
  Mux3 : Mux  Inputs=3
  Mux4 : Mux
  Rate Transition1 : RateTransition  OutPortSampleTime=dt
  Receive1 : xpcrtudplib/Legacy UDP/Receive   ipAddress=000.000.000.000  ipPort=UDP_PORT_DataRecvFromMTM  width=8*17  vblLen=on  sampletime=dtUDP_TeleOpMTM
  Terminator1 : Terminator
  Unpack1 : xpcobsoletelib/Utilities/Unpack   dimensions={1,1,1,1,1,1,1,1,1,1,1,1,1,1,1,1,1}  datatypes={'double' 'double' 'double' 'double' 'double' 'double' 'double' 'double' 'double' 'double' 'double' 'double' 'double' 'double' 'double' 'double' 'double'}  byteAlign=1
  m to mm : Gain  Gain=1000
  sec to msec : Gain  Gain=1000
  MTM : Outport
  wires:
  Unpack1/4 -> Mux3/2  "y"
  Unpack1/9 -> Mux4/4  "q3"
  Unpack1/8 -> Mux4/3  "q2"
  Unpack1/2 -> Discrete Filter3/1  "gripper"
  Mux3/1 -> m to mm/1
  Unpack1/6 -> Mux4/1  "q0"
  Unpack1/7 -> Mux4/2  "q1"
  Unpack1/5 -> Mux3/3  "z"
  Bus Creator1/1 -> Rate Transition1/1
  Receive1/2 -> Terminator1/1
  Receive1/1 -> Unpack1/1
  Unpack1/1 -> Bus Creator1/1  "MSG_Type"
  Mux4/1 -> Discrete Filter1/1
  Unpack1/3 -> Mux3/1  "x"
  m to mm/1 -> Discrete Filter/1
  Rate Transition1/1 -> MTM/1  "MTM"
  Discrete Filter/1 -> MTM Filter/1(current_position), Bus Creator1/3  "position"
  Discrete Filter1/1 -> Bus Creator1/4  "orientation (quat)"
  Unpack1/16 -> Bus Creator1/6  "MTM_time"
  Unpack1/17 -> sec to msec/1
  sec to msec/1 -> Bus Creator1/7  "Delay"
  Unpack1/10 -> Mux1/1  "Fx"
  Unpack1/11 -> Mux1/2  "Fy"
  Unpack1/12 -> Mux1/3  "Fz"
  Unpack1/13 -> Mux1/4  "Mx"
  Unpack1/14 -> Mux1/5  "My"
  Unpack1/15 -> Mux1/6  "Mz"
  Discrete Filter3/1 -> Bus Creator1/2  "gripper"
  Mux1/1 -> Discrete Filter2/1
  Discrete Filter2/1 -> Bus Creator1/5  "MTM_Wrench"
  Discrete Derivative/1 -> Bus Creator1/8  "v_cmd"
  MTM Filter/1(vel_out) -> Discrete Derivative/1

== system xPC_parker/Trajectory Planner/DaVinci MTM port: 2/Davinci Task Ref ==
  MTM : Inport
  x_cmd_prev : Inport  Port=2
  Hybrid_EN : Inport  Port=3
  Bus Creator : BusCreator
  Bus Selector : BusSelector  OutputSignals=MSG_Type,position,orientation (quat),v_cmd
  Constant : Constant  Value=[1 0 0 0]
  N-Sample Switch : dspswit3/N-Sample Switch  N=1  reset=on  TriggerType=Falling edge  Ts=dt
  N-Sample Switch1 : dspswit3/N-Sample Switch  N=1  reset=off  TriggerType=Rising edge  Ts=dt
  R_cmd Delay : UnitDelay  SampleTime=-1
  Task Reference : MATLAB Function  TreatAsAtomicUnit=on
  x_cmd Delay : UnitDelay  SampleTime=-1
  traj : Outport
  wires:
  x_cmd Delay/1 -> N-Sample Switch/2
  x_cmd_prev/1 -> N-Sample Switch/1
  Task Reference/1(x_cmd) -> [x_cmd], x_cmd Delay/1
  Bus Selector/1 -> Task Reference/1(MSG_TYPE)  "<MSG_Type>"
  MTM/1 -> Bus Selector/1
  Bus Selector/2 -> Task Reference/2(x_des)  "<position>"
  N-Sample Switch/1 -> Task Reference/4(xs)
  Task Reference/2(R_cmd) -> [R_cmd], R_cmd Delay/1
  Bus Selector/3 -> Task Reference/3(R_des)  "<orientation (quat)>"
  N-Sample Switch1/1 -> Task Reference/5(Rs)
  Constant/1 -> N-Sample Switch1/1
  R_cmd Delay/1 -> N-Sample Switch1/2
  Task Reference/3(Task_EN) -> [EN]
  [R_cmd] -> Bus Creator/2  "R_cmd"
  Bus Creator/1 -> traj/1
  [x_cmd] -> Bus Creator/1  "x_cmd"
  [EN] -> Bus Creator/3  "Task_EN"
  Bus Selector/4 -> [v_cmd]  "<v_cmd>"
  [v_cmd] -> Bus Creator/4  "v_cmd"
  Hybrid_EN/1 -> N-Sample Switch/3

== system xPC_parker/Trajectory Planner/DaVinci MTM port: 2/UDP_feedback_to_MTM ==
  MTM : Inport
  traj : Inport  Port=2
  force : Inport  Port=3
  pc : Inport  Port=4
  Bus Selector : BusSelector  OutputSignals=Task_EN,R_cmd
  Bus Selector2 : BusSelector  OutputSignals=MSG_Type,MTM_time,Delay
  Demux : Demux  Outputs=17
  Demux1 : Demux  Outputs=2
  Force Filter for MTM : Subsystem
  ForceUnitConv : Gain
  MSG_Decoding : MATLAB Function  TreatAsAtomicUnit=on
  Mux : Mux  Inputs=8
  Pack : xpcobsoletelib/Utilities/Pack   datatypes={'double' 'double' 'double' 'double' 'double' 'double' 'double' 'double' 'double' 'double' 'double' 'double' 'double' 'double' 'double' 'double' 'double'}  byteAlign=1
  Parker_Send : xpcrtudplib/Legacy UDP/Send   ipAddress=255.255.255.255  ipPort=UDP_PORT_DataSend2MTM  localPort=-1  vblLen=off  sampletime=dtUDP_TeleOpMTM
  Rate Transition2 : RateTransition  OutPortSampleTime=dtUDP_TeleOpMTM
  Sum : Sum  Inputs=|++
  TorqueUnitConv : Gain
  mm to m : Gain  Gain=1/1000
  nothing : Constant  Value=0  SampleTime=dt
  wires:
  Pack/1 -> Parker_Send/1
  Mux/1 -> Rate Transition2/1
  Rate Transition2/1 -> Demux/1
  Bus Selector/2 -> Mux/4  "<R_cmd>"
  Demux/1 -> Pack/1
  Demux/2 -> Pack/2
  Demux/3 -> Pack/3
  Demux/4 -> Pack/4
  Demux/5 -> Pack/5
  Demux/6 -> Pack/6
  Demux/7 -> Pack/7
  Demux/8 -> Pack/8
  Demux/9 -> Pack/9
  traj/1 -> Bus Selector/1
  mm to m/1 -> Mux/3
  Demux/10 -> Pack/10
  MTM/1 -> Bus Selector2/1
  Bus Selector2/1 -> MSG_Decoding/1(MSG_Type)  "<MSG_Type>"
  Bus Selector2/2 -> [MTM_time]  "<MTM_time>"
  MSG_Decoding/1(Echo_EN) -> [EchoFlag]
  nothing/1 -> Mux/2
  Bus Selector/1 -> Sum/1  "<Task_EN>"
  [EchoFlag] -> Sum/2
  Sum/1 -> Mux/1
  Bus Selector2/3 -> [TeleOpDelay]  "<Delay>"
  [TeleOpDelay] -> Mux/8
  [MTM_time] -> Mux/7
  force/1 -> Force Filter for MTM/1(V_in)
  Demux1/1 -> ForceUnitConv/1  "Force(N)"
  ForceUnitConv/1 -> Mux/5  "Force(N)"
  Demux1/2 -> TorqueUnitConv/1  "Torque(Nmm)"
  TorqueUnitConv/1 -> Mux/6  "Torque(Nmm)"
  Demux/11 -> Pack/11
  Demux/12 -> Pack/12
  Demux/13 -> Pack/13
  Demux/14 -> Pack/14
  Demux/15 -> Pack/15
  Demux/16 -> Pack/16
  Demux/17 -> Pack/17
  pc/1 -> mm to m/1
  Force Filter for MTM/1(V_Out) -> Demux1/1

== system xPC_parker/Trajectory Planner/Omega7/Feedback_to_omega7 ==
  force : Inport
  Demux1 : Demux
  Demux2 : Demux  Outputs=2
  Force Filter : MATLAB Function  TreatAsAtomicUnit=on
  Is Left Handed : Gain  Gain=Omega7IsLeftHanded
  Mux3 : Mux  Inputs=2
  Pack : xpcobsoletelib/Utilities/Pack   datatypes={'double','double','double','double'}  byteAlign=1
  Rate Transition : RateTransition  OutPortSampleTime=dtOmega7
  "Scope " : slrtlib/Displays and Logging/Scope   scopeno=23  scopetype=Target  autostart=on  viewmode=Numerical  formatstr='%15.6f'  grid=on  ylimits=[0,0]  nosamples=25  noprepostsamples=0  interleave=1  triggermode=FreeRun  triggersignal=1  trigsignalfromport=off  triggerlevel=0.0  triggerslope=Either  triggerscope=1  triggersample=0  filename=data.dat  mode=Lazy  writesize=512  autorestart=off  dynamicfilemode=off  maxwritefilesize=512*1024^2
  Send : xpcrtudplib/Legacy UDP/Send   ipAddress=192.168.1.15  ipPort=19900  localPort=-1  vblLen=off  sampletime=dtOmega7
  Terminator1 : Terminator
  Unit Delay : UnitDelay  SampleTime=-1
  fdelta : Constant  Value=0.002
  fdelta1 : Constant  Value=R_omni
  force feedback filter : Subsystem
  force_UDP_gain : Gain  Gain=[1; 1; 1; 1]
  gripper_force : Constant  Value=-0.8
  wires:
  force/1 -> force feedback filter/1(V_in)
  Pack/1 -> Rate Transition/1
  Demux2/2 -> Terminator1/1
  gripper_force/1 -> Is Left Handed/1
  Rate Transition/1 -> Send/1
  force_UDP_gain/1 -> Force Filter/1(f)
  Force Filter/1(f_out) -> Demux1/1, Unit Delay/1, "Scope "/1
  fdelta/1 -> Force Filter/2(f_delta)
  Unit Delay/1 -> Force Filter/4(f_prev)
  Mux3/1 -> force_UDP_gain/1
  Demux2/1 -> Mux3/1
  force feedback filter/1(V_Out) -> Demux2/1
  Demux1/1 -> Pack/1  "Fx"
  Demux1/2 -> Pack/2  "Fy"
  Demux1/3 -> Pack/3  "Fz"
  Demux1/4 -> Pack/4  "F_gripper"
  Is Left Handed/1 -> Mux3/2
  fdelta1/1 -> Force Filter/3(R_m2s)

== system xPC_parker/Trajectory Planner/Omega7/Omni Task Ref ==
  Omni : Inport
  x_cmd_prev : Inport  Port=2
  Bus Selector : BusSelector  OutputSignals=enable,position,orientation (quat)
  Discrete Derivative : simulink/Discrete/Discrete Derivative  gainval=1.0  ICPrevScaledInput=0.0  InputProcessing=Inherited  OutMin=[]  OutMax=[]  OutDataType=fixdt(1, 16)  OutScaling=2^-10  DoSatur=off
  Gain : Gain  Gain=R_omni  Multiplication=Matrix(K*u)
  N-Sample Switch : dspswit3/N-Sample Switch  N=1  reset=off  TriggerType=Rising edge  Ts=dt
  Task Reference : MATLAB Function  TreatAsAtomicUnit=on
  Terminator : Terminator
  b_R_o : Constant  Value=R_omni
  enOri : Constant  Value=0
  enOri1 : Constant  Value=100
  enOri2 : Constant  Value=dt
  scaling : Constant  Value=omni_scaling
  x_cmd Delay : UnitDelay  SampleTime=-1
  xs Delay : UnitDelay  SampleTime=-1
  x_cmd : Outport
  v_cmd : Outport  Port=2
  wires:
  b_R_o/1 -> Task Reference/1(b_R_o)
  scaling/1 -> Task Reference/2(scaling)
  Omni/1 -> Bus Selector/1
  Task Reference/1(x_cmd) -> x_cmd/1, x_cmd Delay/1
  Task Reference/2(x_s) -> xs Delay/1
  Bus Selector/2 -> Discrete Derivative/1, Task Reference/7(x_tele)  "<position>"
  Bus Selector/3 -> Terminator/1  "<orientation (quat)>"
  xs Delay/1 -> Task Reference/9(x_s_prev)
  N-Sample Switch/1 -> Task Reference/8(x_prev)
  x_cmd_prev/1 -> N-Sample Switch/1
  x_cmd Delay/1 -> N-Sample Switch/2
  Discrete Derivative/1 -> Gain/1
  Gain/1 -> v_cmd/1
  enOri/1 -> Task Reference/4(enOri)
  Bus Selector/1 -> Task Reference/3(enPos)  "<enable>"
  enOri1/1 -> Task Reference/5(vlim)
  enOri2/1 -> Task Reference/6(dt)

== system xPC_parker/Trajectory Planner/Quintic Polynomial/5th Order Polynomial ==
  q des : Inport
  q curr : Inport  Port=2
  enable : Inport  Port=3
  Digital Clock : DigitalClock  SampleTime=dt
  Embedded MATLAB Function : MATLAB Function  TreatAsAtomicUnit=on
  Mux : Mux  Inputs=3
  N-Sample Switch : dspswit3/N-Sample Switch  N=1  reset=off  TriggerType=Rising edge  Ts=dt
  Unit Delay : UnitDelay  SampleTime=dt
  Unit Delay1 : UnitDelay  SampleTime=dt
  Unit Delay2 : UnitDelay  SampleTime=dt
  tf : Constant  Value=5  SampleTime=dt
  q,qd,qdd : Outport
  RecordFlag : Outport  Port=2
  wires:
  Embedded MATLAB Function/4(confn) -> Unit Delay/1
  Unit Delay/1 -> Embedded MATLAB Function/5(conf)
  Embedded MATLAB Function/5(t0n) -> Unit Delay1/1
  Embedded MATLAB Function/6(p0n) -> Unit Delay2/1
  Unit Delay1/1 -> Embedded MATLAB Function/6(t0)
  Digital Clock/1 -> Embedded MATLAB Function/4(tc)
  q des/1 -> Embedded MATLAB Function/1(p_des)
  tf/1 -> Embedded MATLAB Function/3(tf)
  enable/1 -> Embedded MATLAB Function/8(enable)
  Embedded MATLAB Function/1(p) -> Mux/1
  Embedded MATLAB Function/2(pdot) -> Mux/2
  Mux/1 -> q,qd,qdd/1
  Embedded MATLAB Function/3(pdotdot) -> Mux/3
  N-Sample Switch/1 -> Embedded MATLAB Function/7(p0)
  Unit Delay2/1 -> N-Sample Switch/2
  q curr/1 -> [q_cur]
  [q_cur] -> Embedded MATLAB Function/2(p_curr)
  [q_cur] -> N-Sample Switch/1
  Embedded MATLAB Function/7(RECORD) -> RecordFlag/1

== system xPC_parker/Trajectory Planner/Quintic Polynomial/Get_Initial_Condition ==
  q_cur : Inport
  N-Sample Switch : dspswit3/N-Sample Switch  N=1  reset=off  TriggerType=Rising edge  Ts=dt
  Unit Delay : UnitDelay  InitialCondition=zeros(3,1)  SampleTime=-1
  Initial : Outport
  wires:
  N-Sample Switch/1 -> Unit Delay/1, Initial/1
  Unit Delay/1 -> N-Sample Switch/2
  q_cur/1 -> N-Sample Switch/1

== system xPC_parker/Trajectory Planner/Quintic Polynomial/trigger detection ==
  trig : Inport
  Counter : dspswit3/Counter  Direction=Up  CountEvent=Rising edge  CounterSize=User defined  MaxCount=255  InitialCount=0  Output=Count  HitValue=32  ResetInput=off  SamplesPerFrame=1  Ts=1  CntDtype=double  HitDtype=Boolean
  MATLAB Function : MATLAB Function  TreatAsAtomicUnit=on
  Unit Delay : UnitDelay  SampleTime=dt
  enable : Outport
  count : Outport  Port=2
  wires:
  MATLAB Function/1(enable) -> enable/1, Unit Delay/1
  Counter/1 -> count/1, MATLAB Function/1(trig)
  Unit Delay/1 -> MATLAB Function/2(trig_history)
  trig/1 -> Counter/1

== system xPC_parker/Trajectory Planner/Task Enable Logic/PathPlannerLogic ==
  cState : Inport
  Add1 : Sum  Inputs=+++
  Exe State : simulink/Logic and Bit Operations/Compare To Constant  relop===  const=3  OutDataTypeStr=uint8
  Moving to Initial Point : simulink/Logic and Bit Operations/Compare To Constant  relop===  const=1  OutDataTypeStr=uint8
  Waiting State : simulink/Logic and Bit Operations/Compare To Constant  relop===  const=2  OutDataTypeStr=uint8
  TASK_EN : Outport
  wires:
  cState/1 -> Moving to Initial Point/1, Exe State/1, Waiting State/1
  Add1/1 -> TASK_EN/1
  Waiting State/1 -> Add1/2
  Moving to Initial Point/1 -> Add1/1
  Exe State/1 -> Add1/3

== system xPC_parker/Trajectory Planner/Task Input/Hybrid Admittance Controller ==
  note: Hybrid Force / Position Admittance Controller
      | (c) Jason Pile, Long Wang 2014
  x_des : Inport
  f_sensor : Inport  Port=2
  TASK_EN : Inport  Port=3
  x_cur : Inport  Port=4
  Admittance Gain : Gain  Gain=[0 0 0]
  Demux : Demux  Outputs=2
  Discrete-Time Integrator : DiscreteIntegrator  ExternalReset=falling  InitialCondition=zeros(3,1)  SampleTime=-1  LimitOutput=on
  Force Dead Zone : DeadZone  LowerValue=-forceDeadZone  UpperValue=forceDeadZone  SaturateOnIntegerOverflow=on
  Moment Terminator : Terminator
  Mux : Mux  Inputs=2
  N-Sample Enable : dspswit3/N-Sample Enable  N=1  ActiveLevel=Low (0)  reset=off  TriggerType=Rising edge  Ts=dt  DataType=Logical
  Resolved Rates : Subsystem
  Selection Matrix : Gain  Gain=eye(3)-diag([0, 0, 0])  Multiplication=Matrix(K*u)
  Sum : Sum  Inputs=|++
  v_cmd : Outport
  F_adm_scope : Outport  Port=2
  wires:
  f_sensor/1 -> Demux/1
  Demux/2 -> Moment Terminator/1
  Admittance Gain/1 -> [A], Sum/2  "v_f"
  Force Dead Zone/1 -> Admittance Gain/1
  Mux/1 -> F_adm_scope/1
  Sum/1 -> v_cmd/1
  Discrete-Time Integrator/1 -> Mux/2
  Selection Matrix/1 -> [Adm_Force], Force Dead Zone/1
  [Adm_Force] -> Mux/1
  Resolved Rates/1(velocity) -> Sum/1  "v_x"
  [A] -> Discrete-Time Integrator/1
  x_des/1 -> Resolved Rates/2(desired pose)
  x_cur/1 -> Resolved Rates/1(current pose)
  TASK_EN/1 -> Resolved Rates/3(TASK_EN)
  N-Sample Enable/1 -> Discrete-Time Integrator/2
  Demux/1 -> Selection Matrix/1

== system xPC_parker/Trajectory Planner/Task Input/Motion Projector ==
  n : Inport
  Fm : Inport  Port=2
  Projector : MATLAB Function  TreatAsAtomicUnit=on
  v_allowed : Outport
  wires:
  n/1 -> Projector/2(N)
  Projector/1(y) -> v_allowed/1
  Fm/1 -> Projector/1(F)

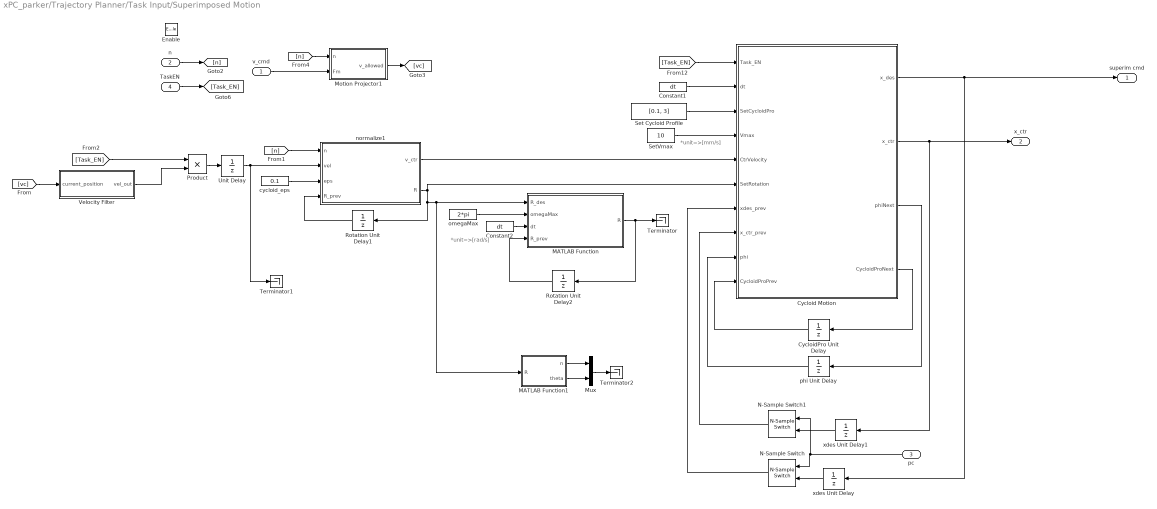
== system xPC_parker/Trajectory Planner/Task Input/Superimposed Motion ==
  note: *unit=>[rad/s]
  note: *unit=>[mm/s]
  v_cmd : Inport
  n : Inport  Port=2
  pc : Inport  Port=3
  TaskEN : Inport  Port=4
  Enable : EnablePort  StatesWhenEnabling=reset
  Constant1 : Constant  Value=dt
  Constant2 : Constant  Value=dt
  Cycloid Motion : MATLAB Function  TreatAsAtomicUnit=on
  CycloidPro Unit Delay : UnitDelay  InitialCondition=[0.5, 5]  SampleTime=-1
  MATLAB Function : MATLAB Function  TreatAsAtomicUnit=on
  MATLAB Function1 : MATLAB Function  TreatAsAtomicUnit=on
  Motion Projector1 : Subsystem  TreatAsAtomicUnit=on
  Mux : Mux  Inputs=2
  N-Sample Switch : dspswit3/N-Sample Switch  N=1  reset=off  TriggerType=Rising edge  Ts=dt
  N-Sample Switch1 : dspswit3/N-Sample Switch  N=1  reset=off  TriggerType=Rising edge  Ts=dt
  Product : Product
  Rotation Unit Delay1 : UnitDelay  InitialCondition=eye(3)  SampleTime=-1
  Rotation Unit Delay2 : UnitDelay  InitialCondition=eye(3)  SampleTime=-1
  Set Cycloid Profile : Constant  Value=[0.1, 3]
  SetVmax : Constant  Value=10
  Terminator : Terminator
  Terminator1 : Terminator
  Terminator2 : Terminator
  Unit Delay : UnitDelay  InitialCondition=zeros(3,1)  SampleTime=-1
  Velocity Filter : Subsystem
  cycloid_eps : Constant  Value=0.1
  normalize1 : MATLAB Function  TreatAsAtomicUnit=on
  omegaMax : Constant  Value=2*pi
  phi Unit Delay : UnitDelay  InitialCondition=pi  SampleTime=-1
  xdes Unit Delay : UnitDelay  InitialCondition=zeros(3,1)  SampleTime=-1
  xdes Unit Delay1 : UnitDelay  InitialCondition=zeros(3,1)  SampleTime=-1
  superim cmd : Outport
  x_ctr : Outport  Port=2
  wires:
  Cycloid Motion/4(CycloidProNext) -> CycloidPro Unit Delay/1
  Constant1/1 -> Cycloid Motion/2(dt)
  Cycloid Motion/3(phiNext) -> phi Unit Delay/1
  Cycloid Motion/1(x_des) -> xdes Unit Delay/1, superim cmd/1
  Set Cycloid Profile/1 -> Cycloid Motion/3(SetCycloidPro)
  normalize1/2(R) -> Cycloid Motion/6(SetRotation), Rotation Unit Delay1/1, MATLAB Function1/1(R), MATLAB Function/1(R_des)
  cycloid_eps/1 -> normalize1/3(eps)
  CycloidPro Unit Delay/1 -> Cycloid Motion/10(CycloidProPrev)
  phi Unit Delay/1 -> Cycloid Motion/9(phi)
  Rotation Unit Delay1/1 -> normalize1/4(R_prev)
  Unit Delay/1 -> Terminator1/1, normalize1/2(vel)
  MATLAB Function/1(R) -> Rotation Unit Delay2/1, Terminator/1
  Rotation Unit Delay2/1 -> MATLAB Function/4(R_prev)
  [n] -> Motion Projector1/1(n)
  v_cmd/1 -> Motion Projector1/2(Fm)
  Motion Projector1/1(v_allowed) -> [vc]
  n/1 -> [n]
  [vc] -> Velocity Filter/1(current_position)
  [n] -> normalize1/1(n)
  normalize1/1(v_ctr) -> Cycloid Motion/5(CtrVelocity)
  Constant2/1 -> MATLAB Function/3(dt)
  omegaMax/1 -> MATLAB Function/2(omegaMax)
  xdes Unit Delay/1 -> N-Sample Switch/2
  N-Sample Switch/1 -> Cycloid Motion/7(xdes_prev)
  pc/1 -> N-Sample Switch1/1, N-Sample Switch/1
  Cycloid Motion/2(x_ctr) -> x_ctr/1, xdes Unit Delay1/1
  N-Sample Switch1/1 -> Cycloid Motion/8(x_ctr_prev)
  xdes Unit Delay1/1 -> N-Sample Switch1/2
  SetVmax/1 -> Cycloid Motion/4(Vmax)
  Mux/1 -> Terminator2/1
  MATLAB Function1/1(n) -> Mux/1
  MATLAB Function1/2(theta) -> Mux/2
  TaskEN/1 -> [Task_EN]
  [Task_EN] -> Cycloid Motion/1(Task_EN)
  Velocity Filter/1(vel_out) -> Product/2
  Product/1 -> Unit Delay/1
  [Task_EN] -> Product/1
